simulink library "BLDC"  (R2012b)
settings: Solver=ode45  StartTime=0.0  StopTime=10.0  RelTol=1e-3
undefined symbols (not defined in the file): fcem_a, fcem_b, fcem_c
libraries: simulink x30, Tools x6
settings Model: Creator=Juliano  LastModifiedBy=h3now

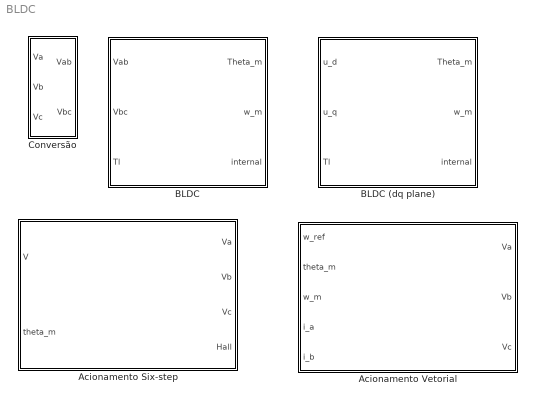
== system BLDC ==
  Acionamento Six-step : Subsystem  mask(Acionamento six-step){P=8}
      mask prompts: P "Número de pólos do motor"
      mask help:
      | Entradas
      | - V: Tensão que será aplicada nas bobinas quando forem comutadas [V]
      | - theta_m: Posição angular do rotor [rad]
      |
      | Saídas
      | - Va: Tensão que deverá ser aplicada na fase a do motor [V]
      | - Vb: Tensão que deverá ser aplicada na fase b do motor [V]
      | - Vc: Tensão que deverá ser aplicada na fase c do motor [V]
      | - Hall: Vetor 3x1 com os sinais logicos de cada sensor hall
  Acionamento Vetorial : Subsystem  mask(Acionamento Vetorial){P=8}
      mask prompts: P "Número de pólos do motor"
      mask help:
      | Entradas
      | - w_ref: Velocidade angular de referência [rpm]
      | - theta_m: Posição angular do rotor [rad]
      | - w_m: Velocidade angular do rotor [rad/s]
      | - i_a: Corrente da fase 'a' do BDLC [A]
      | - i_b: Corrente da fase 'b' do BLDC [A]
      |
      | Saídas
      | - Va: Tensão que deverá ser aplicada na fase a do motor [V]
      | - Vb: Tensão que deverá ser aplicada na fase b do motor [V]
      | - Vc: Tensão que deverá ser aplicada na fase c do motor [V]
  BLDC : Subsystem  mask(Simulador de um motor BLDC){J=1.39e-6, R=10.1/2, L=2.04/2000, P=8, Kt=15.7e-3/1.19, Ke=15.7e-3/1.19, Kd=0, F_stick=0, F_slip=0, default_fcem=on, fcem_a=fcem_a, fcem_b=fcem_b, fcem_c=fcem_c}
      mask prompts: J "Inércia do sistema motor+carga [Kg.m^2]"; R "Resistência por fase [Ohm]"; L "Indutância por fase (descontado o valor da indutância mútua, se for significativo) [Henry]"; P "Número de pólos"; Kt "Constante de torque [Nm/A]"; Ke "Constante de força eletromotriz [V.s] (numericamente igual à constante de torque se utilizar SI)"; Kd "Constante de atrito viscoso"; F_stick "Força máxima de atrito estático"; F_slip "Força de atrito dinâmico"; default_fcem "Utilizar back-emf trapezoidal?"; fcem_a "Lookup table da back-emf fase a"; fcem_b "Lookup table da back-emf fase b"; fcem_c "Lookup table da back-emf fase c"
      mask help:
      | Entradas
      | - Vab: Diferença de potencial entre a fase 'a' e a fase 'b' [V]
      | - Vbc: Diferença de potencial entre a fase 'b' e a fase 'c' [V]
      | - Tl: torque da carga [N.m]
      |
      | Saídas
      | - Theta_m: ângulo do rotor [rad]
      | - w_m: velocidade ângular do rotor [rad/s]
      | - internal: vetor de variáveis internas do simulador:
      |     - FCEM em cada fase [V] (3x1)
      |     - Corrente em cada fase [A] (3x1)
      |     - Torque produzido por cada fase [N.m] (3x1)
      |     - Torque total [N.m] (1x1)
      |     - Torque de atrito [N.m] (1x1)
      mask init:
      | % Se o usuário escolheu utilizar a back-emf padrão, inicializa as variáveis
      | % da lookuptables com valores zerados para não dar erro.
      | if default_fcem == 1
      |     fcem_a = [0,0;1,0];
      |     fcem_b = [0,0;1,0];
      |     fcem_c = [0,0;1,0];
      |     
      | % Se o usuário escolheu especificar qual será a forma da back-emf, checa se
      | % as lookup tables que ele inseriu fazem sentido.
      | else
      |     % Checa se a primeira coluna começa em 0.
      |     if fcem_a(1,1) ~= 0 ||fcem_b(1,1) ~= 0 || fcem_c(1,1) ~= 0
      |         error('A primeira coluna das lookup tables que definem o formato da back-emf devem começar em zero!');
      |     end
      |     % Checa se a primeira coluna termina em 360.
      |     if fcem_a(size(fcem_a,1),1) ~= 360 || fcem_b(size(fcem_b,1),1) ~= 360 || fcem_c(size(fcem_c,1),1) ~= 360
      |         error('A primeira coluna das lookup tables que definem o formato da back-emf deve terminar em 360!');
      |     end
      | end
      mask TypeOptions F_stick: Dinâmica mecânica /Atrito de coulomb/F_stick
      mask TypeOptions F_slip: Dinâmica mecânica /Atrito de coulomb/F_slip
      mask Callback default_fcem:
      | maskStr = get_param(gcb,'MaskValues');
      | 
      | if strcmp(maskStr{10},'on')
      |     set_param(gcb,'MaskVisibilities',{'on';'on';'on';'on';'on';'on';'on';'on';'on';'on';'off';'off';'off'});
      | else
      |     set_param(gcb,'MaskVisibilities',{'on';'on';'on';'on';'on';'on';'on';'on';'on';'on';'on';'on';'on'});
      | end
  BLDC (dq plane) : Subsystem  mask(BLDC Simulator (in dq space coordinates)){J=1.39e-6, R=10.1/2, L=2.04/2000, P=8, Kt=15.7e-3/1.19, Ke=15.7e-3/1.19, Kd=0, F_stick=0, F_slip=0, default_fcem=on, fcem_a=0, fcem_b=0, fcem_c=0}
      mask prompts: J "Inércia do sistema motor+carga [Kg.m^2]"; R "Resistência por Fase [Ohm]"; L "Indutância por fase (descontado o valor da indutância mútua, se for significativo) [Henry]"; P "Número de pólos"; Kt "Constante de torque [N.m/A]"; Ke "Constante de força eletromotriz [V.s]"; Kd "Constante de atrito viscoso"; F_stick "Torque máximo de atrito estático [N.m]"; F_slip "Torque de atrito dinâmico [N.m]"; default_fcem "Utilizar back-emf padrão?"; fcem_a "Forma da back-emf na fase a"; fcem_b "Forma da back-emf na fase b"; fcem_c "Forma da back-emf na fase c"
      mask help:
      | Entradas
      | - u_d: D component of the Vabc voltages projection in the dq plane [V]
      | - u_q: Q component of the Vabc voltages projection in the dq plane [V]
      | - Tl: Load torque [N.m]
      |
      | Saídas
      | - Theta_m: Rotor angle [rad]
      | - w_m: Rotor angular velocity [rad/s]
      | - internal: Vector of internal variables from the simulator:
      |     - Electrical torque: The electrical torque generated by the BLDC
      |     - Currents [2x1]
      |         - i_d: D component of the i_abc currents projection in the dq plane.
      |         - i_q: Q component of the i_abc currents projection in the dq plane.
      |     - Back emfs [2x1]
      |         - e_d: D component of the e_abc back-emfs projection in the dq plane.
      |         - e_q: Q component of the e_abc back_emfs projection in the dq plane.
      |     - Friction Torque: The friction torque acting in the rotor.
      mask init: same as BLDC/BLDC
      mask TypeOptions F_stick: Mechanical model/Atrito de coulomb/F_stick
      mask TypeOptions F_slip: Mechanical model/Atrito de coulomb/F_slip
      mask Callback default_fcem:
      | maskStr = get_param(gcb,'MaskValues');
      | 
      | if strcmp(maskStr{10},'on')
      |     set_param(gcb,'MaskVisibilities',{'on';'on';'on';'on';'on';'on';'on';'on';'on';'on';'off';'off';'off'});
      | else
      |     set_param(gcb,'MaskVisibilities',{'on';'on';'on';'on';'on';'on';'on';'on';'on';'on';'on';'on';'on'});
      | end
  Conversão : Subsystem

== system BLDC/Acionamento Six-step ==
  V : Inport
  theta_m : Inport  Port=2
  Anti-horário : Constant
  Data Type Conversion3 : DataTypeConversion  SaturateOnIntegerOverflow=on  RndMeth=Zero
  Decoder : Subsystem
  Gain : Gain  Gain=P/2
  Inversor : Subsystem
  Sensores Hall : Subsystem
  Va : Outport
  Vb : Outport  Port=2
  Vc : Outport  Port=3
  Hall : Outport  Port=4
  wires:
  theta_m/1 -> Gain/1
  Gain/1 -> Sensores Hall/1(teta_e)
  Decoder/1(Gates) -> Inversor/1(Gates)
  Anti-horário/1 -> Decoder/2(Sentido de rotação)
  V/1 -> Inversor/2(Vcc)
  Sensores Hall/1(Hall) -> Hall/1, Data Type Conversion3/1  "Hall"
  Data Type Conversion3/1 -> Decoder/1("Hall ")
  Inversor/1(Va) -> Va/1
  Inversor/2(Vb) -> Vb/1
  Inversor/3(Vc) -> Vc/1

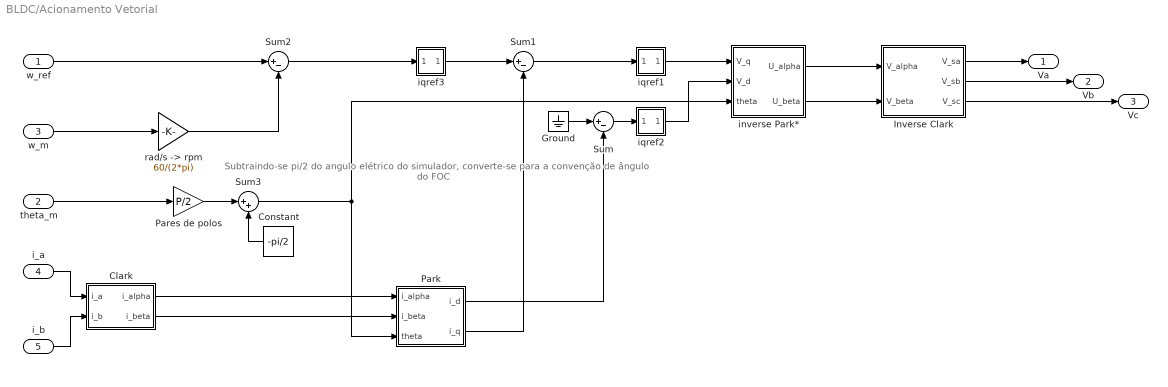
== system BLDC/Acionamento Vetorial ==
  note: Subtraindo-se pi/2 do angulo elétrico
      | do simulador, converte-se para a
      | convenção de ângulo do FOC
  w_ref : Inport
  theta_m : Inport  Port=2
  w_m : Inport  Port=3
  i_a : Inport  Port=4
  i_b : Inport  Port=5
  Clark : Subsystem
  Constant : Constant  Value=-pi/2
  Ground : Ground
  Inverse Clark : Subsystem
  Pares de polos : Gain  Gain=P/2
  Park : Subsystem
  Sum : Sum  Inputs=|+-
  Sum1 : Sum  Inputs=|+-
  Sum2 : Sum  Inputs=|+-
  Sum3 : Sum  Inputs=|++
  inverse Park* : Subsystem
  iqref1 : Subsystem  mask(PI Controller){I=0.5, P=1, sat=[-500, 500]}
      mask prompts: I "Integral"; P "Proportional:"; sat "Minimum and maximum outputs:"
      mask init:
      | min=sat(1);max=sat(2);
      mask Display: disp('PI')
  iqref2 : Subsystem  mask(PI Controller){I=5, P=10, sat=[-500, 500]}
      mask prompts: I "Integral"; P "Proportional:"; sat "Minimum and maximum outputs:"
      mask init:
      | min=sat(1);max=sat(2);
      mask Display: disp('PI')
  iqref3 : Subsystem  mask(PI Controller){I=0.1, P=0.1, sat=[-500, 500]}
      mask prompts: I "Integral"; P "Proportional:"; sat "Minimum and maximum outputs:"
      mask init:
      | min=sat(1);max=sat(2);
      mask Display: disp('PI')
  "rad/s -> rpm" : Gain  Gain=60/(2*pi)
  Va : Outport
  Vb : Outport  Port=2
  Vc : Outport  Port=3
  wires:
  theta_m/1 -> Pares de polos/1
  Pares de polos/1 -> Sum3/1
  Constant/1 -> Sum3/2
  w_ref/1 -> Sum2/1
  i_b/1 -> Clark/2(i_b)
  Sum1/1 -> iqref1/1(In_1)
  Inverse Clark/2(V_sb) -> Vb/1
  Sum2/1 -> iqref3/1(In_1)
  iqref3/1(Out_1) -> Sum1/1
  Inverse Clark/1(V_sa) -> Va/1
  Inverse Clark/3(V_sc) -> Vc/1
  i_a/1 -> Clark/1(i_a)
  iqref1/1(Out_1) -> inverse Park*/1(V_q)
  "rad/s -> rpm"/1 -> Sum2/2
  Park/2(i_q) -> Sum1/2
  Sum3/1 -> inverse Park*/3(theta), Park/3(theta)
  iqref2/1(Out_1) -> inverse Park*/2(V_d)
  w_m/1 -> "rad/s -> rpm"/1
  Ground/1 -> Sum/1
  Park/1(i_d) -> Sum/2
  Sum/1 -> iqref2/1(In_1)
  Clark/2(i_beta) -> Park/2(i_beta)
  Clark/1(i_alpha) -> Park/1(i_alpha)
  inverse Park*/1(U_alpha) -> Inverse Clark/1(V_alpha)
  inverse Park*/2(U_beta) -> Inverse Clark/2(V_beta)

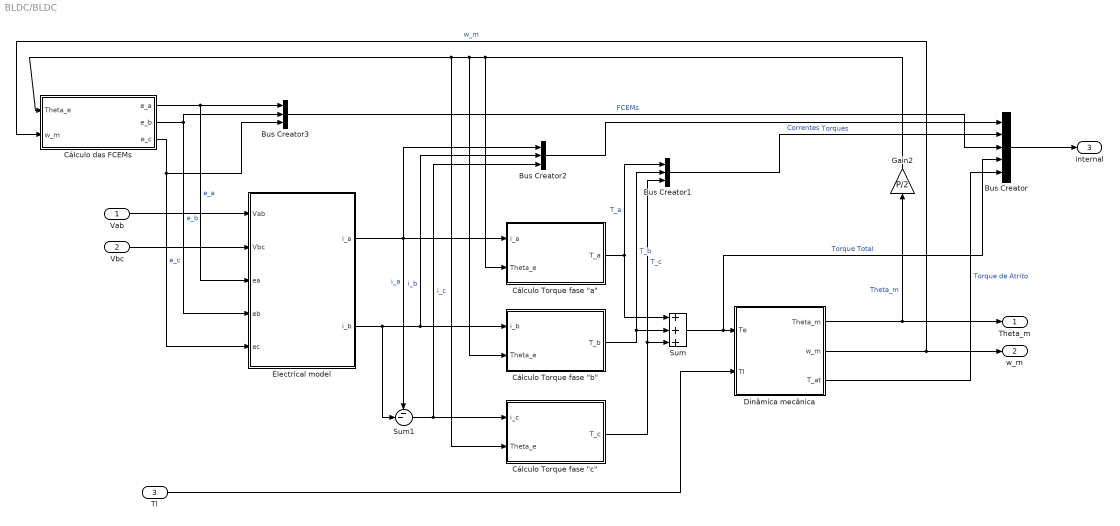
== system BLDC/BLDC ==
  Vab : Inport
  Vbc : Inport  Port=2
  Tl : Inport  Port=3
  Bus Creator : BusCreator  Inputs=5
  Bus Creator1 : BusCreator  Inputs=3
  Bus Creator2 : BusCreator  Inputs=3
  Bus Creator3 : BusCreator  Inputs=3
  "Cálculo Torque fase \"a\"" : Subsystem
  "Cálculo Torque fase \"b\"" : Subsystem
  "Cálculo Torque fase \"c\"" : Subsystem
  Cálculo das FCEMs : Subsystem
  "Dinâmica mecânica " : Subsystem
  Electrical model : Subsystem
  Gain2 : Gain  Gain=P/2
  Sum : Sum  Inputs=+++
  Sum1 : Sum  Inputs=--|
  Theta_m : Outport
  w_m : Outport  Port=2
  internal : Outport  Port=3
  wires:
  Gain2/1 -> "Cálculo Torque fase \"b\""/2(Theta_e), Cálculo das FCEMs/1(Theta_e), "Cálculo Torque fase \"c\""/2(Theta_e), "Cálculo Torque fase \"a\""/2(Theta_e)
  Tl/1 -> "Dinâmica mecânica "/2(Tl)
  "Dinâmica mecânica "/2(w_m) -> Cálculo das FCEMs/2(w_m), w_m/1  "w_m"
  "Dinâmica mecânica "/1(Theta_m) -> Gain2/1, Theta_m/1  "Theta_m"
  Sum/1 -> Bus Creator/4, "Dinâmica mecânica "/1(Te)  "Torque Total"
  "Cálculo Torque fase \"c\""/1(T_c) -> Bus Creator1/3, Sum/3  "T_c"
  "Cálculo Torque fase \"b\""/1(T_b) -> Bus Creator1/2, Sum/2  "T_b"
  "Cálculo Torque fase \"a\""/1(T_a) -> Bus Creator1/1, Sum/1  "T_a"
  Sum1/1 -> "Cálculo Torque fase \"c\""/1(i_c), Bus Creator2/3  "i_c"
  Electrical model/2(i_b) -> "Cálculo Torque fase \"b\""/1(i_b), Bus Creator2/2, Sum1/2  "i_b"
  Electrical model/1(i_a) -> "Cálculo Torque fase \"a\""/1(i_a), Bus Creator2/1, Sum1/1  "i_a"
  Vbc/1 -> Electrical model/2(Vbc)
  Cálculo das FCEMs/3(e_c) -> Electrical model/5(ec), Bus Creator3/3  "e_c"
  Cálculo das FCEMs/2(e_b) -> Electrical model/4(eb), Bus Creator3/2  "e_b"
  Cálculo das FCEMs/1(e_a) -> Electrical model/3(ea), Bus Creator3/1  "e_a"
  Bus Creator/1 -> internal/1
  Bus Creator3/1 -> Bus Creator/3  "FCEMs"
  Bus Creator2/1 -> Bus Creator/1  "Correntes"
  Bus Creator1/1 -> Bus Creator/2  "Torques"
  Vab/1 -> Electrical model/1(Vab)
  "Dinâmica mecânica "/3(T_at) -> Bus Creator/5  "Torque de Atrito"

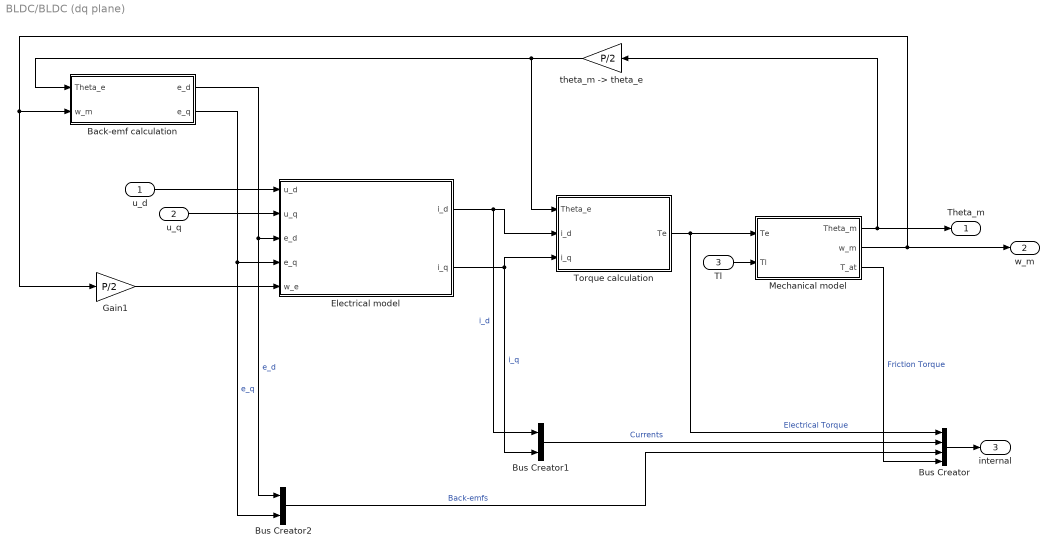
== system BLDC/BLDC (dq plane) ==
  u_d : Inport
  u_q : Inport  Port=2
  Tl : Inport  Port=3
  Back-emf calculation : Subsystem
  Bus Creator : BusCreator
  Bus Creator1 : BusCreator  Inputs=2
  Bus Creator2 : BusCreator  Inputs=2
  Electrical model : Subsystem
  Gain1 : Gain  Gain=P/2
  Mechanical model : Subsystem
  Torque calculation : Subsystem
  "theta_m -> theta_e" : Gain  Gain=P/2
  Theta_m : Outport
  w_m : Outport  Port=2
  internal : Outport  Port=3
  wires:
  Back-emf calculation/2(e_q) -> Bus Creator2/2, Electrical model/4(e_q)  "e_q"
  u_q/1 -> Electrical model/2(u_q)
  Tl/1 -> Mechanical model/2(Tl)
  Mechanical model/2(w_m) -> w_m/1, Back-emf calculation/2(w_m), Gain1/1
  Mechanical model/1(Theta_m) -> "theta_m -> theta_e"/1, Theta_m/1
  "theta_m -> theta_e"/1 -> Torque calculation/1(Theta_e), Back-emf calculation/1(Theta_e)
  Gain1/1 -> Electrical model/5(w_e)
  u_d/1 -> Electrical model/1(u_d)
  Back-emf calculation/1(e_d) -> Electrical model/3(e_d), Bus Creator2/1  "e_d"
  Electrical model/1(i_d) -> Bus Creator1/1, Torque calculation/2(i_d)  "i_d"
  Electrical model/2(i_q) -> Bus Creator1/2, Torque calculation/3(i_q)  "i_q"
  Torque calculation/1(Te) -> Bus Creator/1, Mechanical model/1(Te)  "Electrical Torque"
  Bus Creator1/1 -> Bus Creator/2  "Currents"
  Bus Creator2/1 -> Bus Creator/3  "Back-emfs"
  Bus Creator/1 -> internal/1
  Mechanical model/3(T_at) -> Bus Creator/4  "Friction Torque"

== system BLDC/Conversão ==
  Va : Inport
  Vb : Inport  Port=2
  Vc : Inport  Port=3
  Sum : Sum  Inputs=|+-
  Sum1 : Sum  Inputs=|+-
  Vab : Outport
  Vbc : Outport  Port=2
  wires:
  Va/1 -> Sum/1
  Sum/1 -> Vab/1
  Vb/1 -> Sum1/1, Sum/2
  Vc/1 -> Sum1/2
  Sum1/1 -> Vbc/1

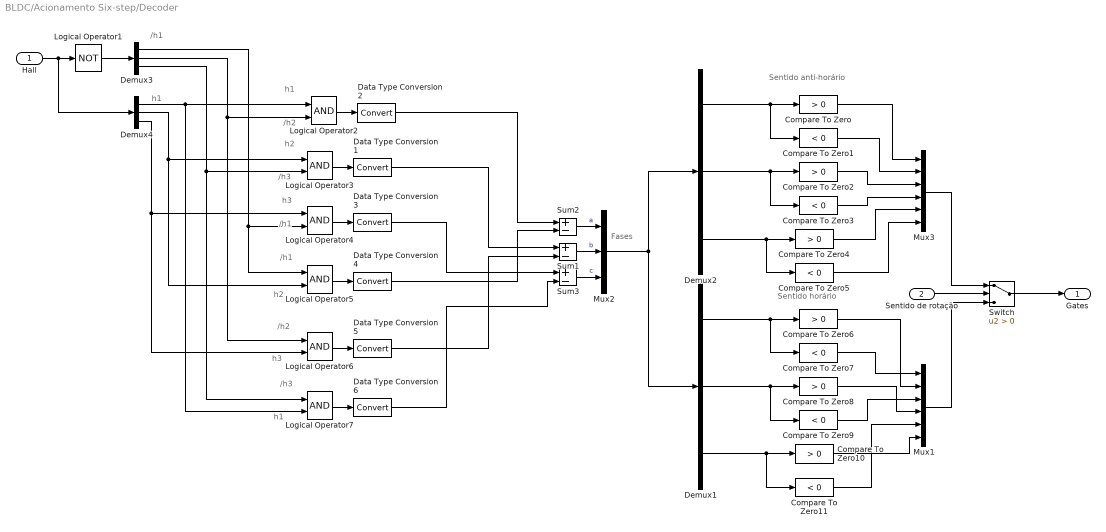
== system BLDC/Acionamento Six-step/Decoder ==
  note: Fases
  note: Sentido horário
  note: Sentido anti-horário
  note: h1
  note: /h3
  note: h3
  note: /h2
  note: h2
  note: /h1
  note: /h1
  note: h3
  note: /h3
  note: h2
  note: /h2
  note: h1
  note: h1
  note: /h1
  "Hall " : Inport
  Sentido de rotação : Inport  Port=2
  Compare To Zero{,2,4,6,8,10} (6 alike) : simulink/Logic and Bit Operations/Compare To Zero  relop=>  OutDataTypeStr=boolean  ZeroCross=off
  Compare To Zero{1,3,5,7,9,11} (6 alike) : simulink/Logic and Bit Operations/Compare To Zero  relop=<  OutDataTypeStr=boolean  ZeroCross=off
  Data Type Conversion{1..6} (6 alike) : DataTypeConversion
  Demux{1..4} (4 alike) : Demux  Outputs=3
  Logical Operator1 : Logic  Operator=NOT  AllPortsSameDT=off  OutDataTypeStr=boolean
  Logical Operator{2..7} (6 alike) : Logic  AllPortsSameDT=off  OutDataTypeStr=boolean
  Mux1 : Mux  Inputs=6
  Mux2 : Mux  Inputs=3
  Mux3 : Mux  Inputs=6
  Sum1 : Sum  Inputs=+-  OutDataTypeStr=double
  Sum2 : Sum  Inputs=+-  OutDataTypeStr=double
  Sum3 : Sum  Inputs=+-  OutDataTypeStr=double
  Switch : Switch  Criteria=u2 > Threshold
  Gates : Outport
  wires:
  Mux2/1 -> Demux1/1, Demux2/1
  Data Type Conversion6/1 -> Sum3/2
  Data Type Conversion3/1 -> Sum3/1
  Data Type Conversion5/1 -> Sum1/2
  Data Type Conversion1/1 -> Sum1/1
  Data Type Conversion4/1 -> Sum2/2
  Data Type Conversion2/1 -> Sum2/1
  Logical Operator7/1 -> Data Type Conversion6/1
  Logical Operator6/1 -> Data Type Conversion5/1
  Logical Operator5/1 -> Data Type Conversion4/1
  Logical Operator4/1 -> Data Type Conversion3/1
  Logical Operator3/1 -> Data Type Conversion1/1
  Sum3/1 -> Mux2/3  "c"
  Sum1/1 -> Mux2/2  "b"
  Sum2/1 -> Mux2/1  "a"
  Logical Operator2/1 -> Data Type Conversion2/1
  Demux3/1 -> Logical Operator5/1, Logical Operator4/2
  Demux3/2 -> Logical Operator6/1, Logical Operator2/2
  Demux3/3 -> Logical Operator7/1, Logical Operator3/2
  Demux4/1 -> Logical Operator7/2, Logical Operator2/1
  Demux4/2 -> Logical Operator5/2, Logical Operator3/1
  Demux4/3 -> Logical Operator6/2, Logical Operator4/1
  Logical Operator1/1 -> Demux3/1
  "Hall "/1 -> Demux4/1, Logical Operator1/1
  Compare To Zero10/1 -> Mux1/6
  Compare To Zero11/1 -> Mux1/5
  Compare To Zero8/1 -> Mux1/4
  Compare To Zero9/1 -> Mux1/3
  Compare To Zero6/1 -> Mux1/2
  Compare To Zero7/1 -> Mux1/1
  Switch/1 -> Gates/1
  Mux1/1 -> Switch/3
  Sentido de rotação/1 -> Switch/2
  Mux3/1 -> Switch/1
  Demux1/3 -> Compare To Zero11/1, Compare To Zero10/1
  Demux1/2 -> Compare To Zero9/1, Compare To Zero8/1
  Demux1/1 -> Compare To Zero7/1, Compare To Zero6/1
  Compare To Zero5/1 -> Mux3/6
  Compare To Zero4/1 -> Mux3/5
  Compare To Zero3/1 -> Mux3/4
  Compare To Zero2/1 -> Mux3/3
  Compare To Zero1/1 -> Mux3/2
  Compare To Zero/1 -> Mux3/1
  Demux2/3 -> Compare To Zero5/1, Compare To Zero4/1
  Demux2/2 -> Compare To Zero3/1, Compare To Zero2/1
  Demux2/1 -> Compare To Zero1/1, Compare To Zero/1

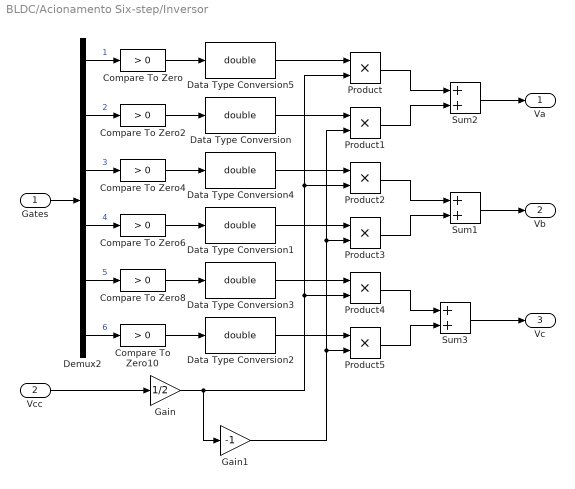
== system BLDC/Acionamento Six-step/Inversor ==
  Gates : Inport
  Vcc : Inport  Port=2
  Compare To Zero : simulink/Logic and Bit Operations/Compare To Zero  relop=>  OutDataTypeStr=uint8  ZeroCross=off
  Compare To Zero{2,6,8,10} (4 alike) : simulink/Logic and Bit Operations/Compare To Zero  relop=>  OutDataTypeStr=boolean  ZeroCross=off
  Compare To Zero4 : simulink/Logic and Bit Operations/Compare To Zero  relop=>  OutDataTypeStr=uint8  ZeroCross=off
  Data Type Conversion{,1..5} (6 alike) : DataTypeConversion  OutDataTypeStr=double
  Demux2 : Demux  Outputs=6
  Gain : Gain  Gain=1/2
  Gain1 : Gain  Gain=-1
  Product{,1..5} (6 alike) : Product  RndMeth=Zero
  Sum1 : Sum  SaturateOnIntegerOverflow=on
  Sum2 : Sum  SaturateOnIntegerOverflow=on
  Sum3 : Sum  SaturateOnIntegerOverflow=on
  Va : Outport
  Vb : Outport  Port=2
  Vc : Outport  Port=3
  wires:
  Vcc/1 -> Gain/1
  Sum1/1 -> Vb/1
  Sum3/1 -> Vc/1
  Sum2/1 -> Va/1
  Gates/1 -> Demux2/1
  Demux2/1 -> Compare To Zero/1  "1"
  Demux2/2 -> Compare To Zero2/1  "2"
  Demux2/3 -> Compare To Zero4/1  "3"
  Demux2/4 -> Compare To Zero6/1  "4"
  Demux2/5 -> Compare To Zero8/1  "5"
  Demux2/6 -> Compare To Zero10/1  "6"
  Compare To Zero/1 -> Data Type Conversion5/1
  Compare To Zero2/1 -> Data Type Conversion/1
  Compare To Zero4/1 -> Data Type Conversion4/1
  Compare To Zero6/1 -> Data Type Conversion1/1
  Compare To Zero8/1 -> Data Type Conversion3/1
  Compare To Zero10/1 -> Data Type Conversion2/1
  Product/1 -> Sum2/1
  Product1/1 -> Sum2/2
  Product2/1 -> Sum1/1
  Product3/1 -> Sum1/2
  Product4/1 -> Sum3/1
  Product5/1 -> Sum3/2
  Data Type Conversion2/1 -> Product5/1
  Data Type Conversion3/1 -> Product4/1
  Data Type Conversion1/1 -> Product3/1
  Data Type Conversion4/1 -> Product2/1
  Data Type Conversion/1 -> Product1/1
  Data Type Conversion5/1 -> Product/1
  Gain1/1 -> Product5/2, Product3/2, Product1/2
  Gain/1 -> Gain1/1, Product4/2, Product2/2, Product/2

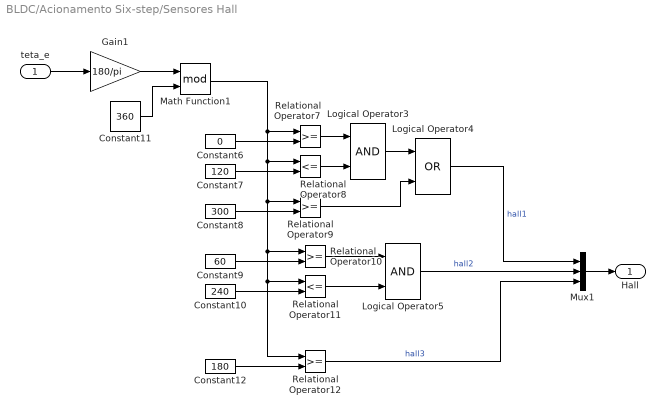
== system BLDC/Acionamento Six-step/Sensores Hall ==
  teta_e : Inport
  Constant10 : Constant  Value=240
  Constant11 : Constant  Value=360
  Constant12 : Constant  Value=180
  Constant6 : Constant  Value=0
  Constant7 : Constant  Value=120
  Constant8 : Constant  Value=300
  Constant9 : Constant  Value=60
  Gain1 : Gain  Gain=180/pi
  Logical Operator3 : Logic  AllPortsSameDT=off  OutDataTypeStr=boolean
  Logical Operator4 : Logic  Operator=OR  AllPortsSameDT=off  OutDataTypeStr=boolean
  Logical Operator5 : Logic  AllPortsSameDT=off  OutDataTypeStr=boolean
  Math Function1 : Math  Operator=mod  SaturateOnIntegerOverflow=on
  Mux1 : Mux  Inputs=3
  Relational Operator{7,9..10,12} (4 alike) : RelationalOperator  InputSameDT=on
  Relational Operator11 : RelationalOperator  Operator=<=  InputSameDT=on
  Relational Operator8 : RelationalOperator  Operator=<=  InputSameDT=on
  Hall : Outport
  wires:
  teta_e/1 -> Gain1/1
  Constant6/1 -> Relational Operator7/2
  Constant7/1 -> Relational Operator8/2
  Constant8/1 -> Relational Operator9/2
  Relational Operator9/1 -> Logical Operator4/2
  Logical Operator3/1 -> Logical Operator4/1
  Relational Operator7/1 -> Logical Operator3/1
  Relational Operator8/1 -> Logical Operator3/2
  Relational Operator10/1 -> Logical Operator5/1
  Relational Operator11/1 -> Logical Operator5/2
  Constant9/1 -> Relational Operator10/2
  Constant10/1 -> Relational Operator11/2
  Constant12/1 -> Relational Operator12/2
  Mux1/1 -> Hall/1
  Logical Operator4/1 -> Mux1/1  "hall1"
  Logical Operator5/1 -> Mux1/2  "hall2"
  Relational Operator12/1 -> Mux1/3  "hall3"
  Gain1/1 -> Math Function1/1
  Constant11/1 -> Math Function1/2
  Math Function1/1 -> Relational Operator8/1, Relational Operator9/1, Relational Operator10/1, Relational Operator11/1, Relational Operator12/1, Relational Operator7/1

== system BLDC/Acionamento Vetorial/Clark ==
  i_a : Inport
  i_b : Inport  Port=2
  Add : Sum
  Gain : Gain  Gain=2
  Gain1 : Gain  Gain=1/sqrt(3)
  i_alpha : Outport
  i_beta : Outport  Port=2
  wires:
  Gain1/1 -> i_beta/1
  Add/1 -> Gain1/1
  Gain/1 -> Add/2
  i_b/1 -> Gain/1
  i_a/1 -> Add/1, i_alpha/1

== system BLDC/Acionamento Vetorial/Inverse Clark ==
  V_alpha : Inport
  V_beta : Inport  Port=2
  Add : Sum  Inputs=-+
  Add1 : Sum  Inputs=--
  Gain : Gain  Gain=0.5
  Gain1 : Gain  Gain=sqrt(3)
  Gain2 : Gain  Gain=0.5
  V_sa : Outport
  V_sb : Outport  Port=2
  V_sc : Outport  Port=3
  wires:
  Gain1/1 -> Add1/1, Add/2
  V_beta/1 -> Gain1/1
  Gain2/1 -> V_sc/1
  Add1/1 -> Gain2/1
  Gain/1 -> V_sb/1
  Add/1 -> Gain/1
  V_alpha/1 -> V_sa/1, Add1/2, Add/1

== system BLDC/Acionamento Vetorial/Park ==
  i_alpha : Inport
  i_beta : Inport  Port=2
  theta : Inport  Port=3
  Add : Sum
  Add1 : Sum  Inputs=-+
  Product : Product  RndMeth=Zero
  Product1 : Product  RndMeth=Zero
  Trigonometric Function : Trigonometry  OutputSignalType=real
  Trigonometric Function1 : Trigonometry  Operator=cos  OutputSignalType=real
  i_d : Outport
  i_q : Outport  Port=2
  wires:
  Add1/1 -> i_q/1
  Product1/1 -> Add1/2, Add/2
  Product/1 -> Add1/1, Add/1
  i_alpha/1 -> Product1/2
  Trigonometric Function1/1 -> Product1/1
  Add/1 -> i_d/1
  Trigonometric Function/1 -> Product/2
  i_beta/1 -> Product/1
  theta/1 -> Trigonometric Function1/1, Trigonometric Function/1

== system BLDC/Acionamento Vetorial/inverse Park* ==
  note: U_alpha = V_d*cos(theta) - V_q*sin(theta)
      | U_beta = V_d*sin(theta) + V_q*cos(theta)
  V_q : Inport
  V_d : Inport  Port=2
  theta : Inport  Port=3
  Add : Sum
  Add1 : Sum  Inputs=-+
  Gain : Gain
  Gain1 : Gain
  Product{,1..3} (4 alike) : Product  RndMeth=Zero
  Trigonometric Function : Trigonometry  OutputSignalType=real
  Trigonometric Function1 : Trigonometry  Operator=cos  OutputSignalType=real
  U_alpha : Outport
  U_beta : Outport  Port=2
  wires:
  Gain1/1 -> U_alpha/1
  Add1/1 -> Gain1/1
  Gain/1 -> U_beta/1
  Add/1 -> Gain/1
  Product3/1 -> Add1/1
  Product2/1 -> Add1/2
  Product1/1 -> Add/2
  Product/1 -> Add/1
  Trigonometric Function/1 -> Product3/1, Product1/1
  V_d/1 -> Product2/2, Product1/2
  Trigonometric Function1/1 -> Product2/1, Product/2
  V_q/1 -> Product3/2, Product/1
  theta/1 -> Trigonometric Function/1, Trigonometric Function1/1

== system BLDC/Acionamento Vetorial/iqref1 ==
  In_1 : Inport
  Integral : TransferFcn  Numerator=[I]  Denominator=[1 0]
  Proportional : Gain  Gain=P  SaturateOnIntegerOverflow=on  OutDataTypeStr=Inherit: Same as input  ParamDataTypeStr=Inherit: Same as input
  Saturation : Saturate  UpperLimit=max  LowerLimit=min
  Sum : Sum  SaturateOnIntegerOverflow=on  InputSameDT=on  OutDataTypeStr=Inherit: Same as first input
  Out_1 : Outport  InitialOutput=0
  wires:
  Integral/1 -> Sum/2
  In_1/1 -> Integral/1, Proportional/1
  Proportional/1 -> Sum/1
  Sum/1 -> Saturation/1
  Saturation/1 -> Out_1/1

== system BLDC/Acionamento Vetorial/iqref2 ==
  In_1 : Inport
  Integral : TransferFcn  Numerator=[I]  Denominator=[1 0]
  Proportional : Gain  Gain=P  SaturateOnIntegerOverflow=on  OutDataTypeStr=Inherit: Same as input  ParamDataTypeStr=Inherit: Same as input
  Saturation : Saturate  UpperLimit=max  LowerLimit=min
  Sum : Sum  SaturateOnIntegerOverflow=on  InputSameDT=on  OutDataTypeStr=Inherit: Same as first input
  Out_1 : Outport  InitialOutput=0
  wires:
  Integral/1 -> Sum/2
  In_1/1 -> Integral/1, Proportional/1
  Proportional/1 -> Sum/1
  Sum/1 -> Saturation/1
  Saturation/1 -> Out_1/1

== system BLDC/Acionamento Vetorial/iqref3 ==
  In_1 : Inport
  Integral : TransferFcn  Numerator=[I]  Denominator=[1 0]
  Proportional : Gain  Gain=P  SaturateOnIntegerOverflow=on  OutDataTypeStr=Inherit: Same as input  ParamDataTypeStr=Inherit: Same as input
  Saturation : Saturate  UpperLimit=max  LowerLimit=min
  Sum : Sum  SaturateOnIntegerOverflow=on  InputSameDT=on  OutDataTypeStr=Inherit: Same as first input
  Out_1 : Outport  InitialOutput=0
  wires:
  Integral/1 -> Sum/2
  In_1/1 -> Proportional/1, Integral/1
  Proportional/1 -> Sum/1
  Sum/1 -> Saturation/1
  Saturation/1 -> Out_1/1

== system BLDC/BLDC/Cálculo Torque fase "a" ==
  i_a : Inport
  Theta_e : Inport  Port=2
  Constant1 : Constant  Value=360
  Gain : Gain  Gain=Kt/2
  Gain1 : Gain  Gain=180/pi
  Math Function1 : Math  Operator=mod  SaturateOnIntegerOverflow=on
  Product : Product  RndMeth=Zero
  forma back-emf a : Subsystem
  T_a : Outport
  wires:
  Constant1/1 -> Math Function1/2
  Gain1/1 -> Math Function1/1
  Product/1 -> T_a/1
  forma back-emf a/1(e_a) -> Product/1
  Theta_e/1 -> Gain1/1
  Math Function1/1 -> forma back-emf a/1(theta)
  Gain/1 -> Product/2
  i_a/1 -> Gain/1

== system BLDC/BLDC/Cálculo Torque fase "b" ==
  i_b : Inport
  Theta_e : Inport  Port=2
  Constant1 : Constant  Value=360
  Gain : Gain  Gain=Kt/2
  Gain1 : Gain  Gain=180/pi
  Math Function1 : Math  Operator=mod  SaturateOnIntegerOverflow=on
  Product : Product  RndMeth=Zero
  forma back-emf b : Subsystem
  T_b : Outport
  wires:
  Constant1/1 -> Math Function1/2
  Gain1/1 -> Math Function1/1
  i_b/1 -> Gain/1
  Gain/1 -> Product/2
  Math Function1/1 -> forma back-emf b/1(theta)
  Theta_e/1 -> Gain1/1
  forma back-emf b/1(e_b) -> Product/1
  Product/1 -> T_b/1

== system BLDC/BLDC/Cálculo Torque fase "c" ==
  i_c : Inport
  Theta_e : Inport  Port=2
  Constant1 : Constant  Value=360
  Gain : Gain  Gain=Kt/2
  Gain1 : Gain  Gain=180/pi
  Math Function1 : Math  Operator=mod  SaturateOnIntegerOverflow=on
  Product : Product  RndMeth=Zero
  forma back-emf c : Subsystem
  T_c : Outport
  wires:
  Constant1/1 -> Math Function1/2
  Gain1/1 -> Math Function1/1
  Product/1 -> T_c/1
  forma back-emf c/1(e_c) -> Product/1
  Theta_e/1 -> Gain1/1
  Math Function1/1 -> forma back-emf c/1(theta)
  Gain/1 -> Product/2
  i_c/1 -> Gain/1

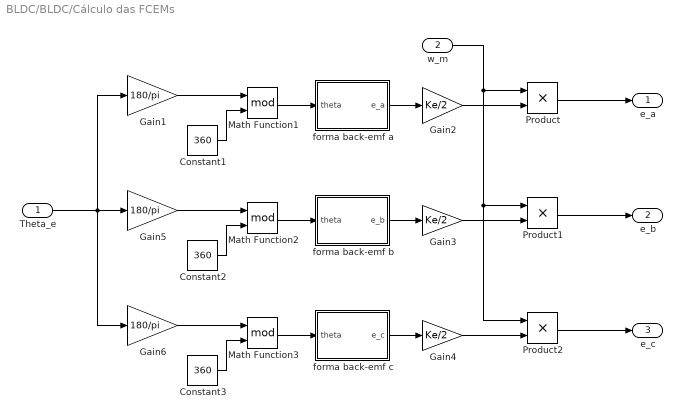
== system BLDC/BLDC/Cálculo das FCEMs ==
  Theta_e : Inport
  w_m : Inport  Port=2
  Constant1 : Constant  Value=360
  Constant2 : Constant  Value=360
  Constant3 : Constant  Value=360
  Gain1 : Gain  Gain=180/pi
  Gain2 : Gain  Gain=Ke/2
  Gain3 : Gain  Gain=Ke/2
  Gain4 : Gain  Gain=Ke/2
  Gain5 : Gain  Gain=180/pi
  Gain6 : Gain  Gain=180/pi
  Math Function1 : Math  Operator=mod  SaturateOnIntegerOverflow=on
  Math Function2 : Math  Operator=mod  SaturateOnIntegerOverflow=on
  Math Function3 : Math  Operator=mod  SaturateOnIntegerOverflow=on
  Product : Product  RndMeth=Zero
  Product1 : Product  RndMeth=Zero
  Product2 : Product  RndMeth=Zero
  forma back-emf a : Subsystem
  forma back-emf b : Subsystem
  forma back-emf c : Subsystem
  e_a : Outport
  e_b : Outport  Port=2
  e_c : Outport  Port=3
  wires:
  Constant3/1 -> Math Function3/2
  Constant2/1 -> Math Function2/2
  Constant1/1 -> Math Function1/2
  Product/1 -> e_a/1
  Product1/1 -> e_b/1
  Theta_e/1 -> Gain5/1, Gain1/1, Gain6/1
  Product2/1 -> e_c/1
  Gain2/1 -> Product/2
  w_m/1 -> Product/1, Product1/1, Product2/1
  Gain3/1 -> Product1/2
  Gain4/1 -> Product2/2
  Gain1/1 -> Math Function1/1
  Gain5/1 -> Math Function2/1
  Gain6/1 -> Math Function3/1
  Math Function1/1 -> forma back-emf a/1(theta)
  forma back-emf a/1(e_a) -> Gain2/1
  Math Function2/1 -> forma back-emf b/1(theta)
  forma back-emf b/1(e_b) -> Gain3/1
  Math Function3/1 -> forma back-emf c/1(theta)
  forma back-emf c/1(e_c) -> Gain4/1

== system BLDC/BLDC/Dinâmica mecânica  ==
  Te : Inport
  Tl : Inport  Port=2
  Atrito de coulomb : Tools/Coulomb Friction  F_stick=F_stick  F_slip=F_slip
  Gain : Gain  Gain=1/J
  Gain1 : Gain  Gain=Kd
  Integrator : Integrator  ExternalReset=rising  ShowStatePort=on
  Integrator1 : Integrator
  Sum1 : Sum  Inputs=+--
  Sum2 : Sum  Inputs=+-
  Theta_m : Outport
  w_m : Outport  Port=2
  T_at : Outport  Port=3
  wires:
  Integrator1/1 -> Theta_m/1
  Tl/1 -> Sum1/2
  Gain1/1 -> Sum1/3
  Te/1 -> Sum1/1
  Integrator/1 -> Atrito de coulomb/3, w_m/1, Integrator1/1, Gain1/1
  Gain/1 -> Integrator/1
  Sum2/1 -> Gain/1
  Sum1/1 -> Sum2/1, Atrito de coulomb/1
  Atrito de coulomb/1 -> T_at/1, Sum2/2
  Atrito de coulomb/2 -> Integrator/2
  Integrator/State -> Atrito de coulomb/2

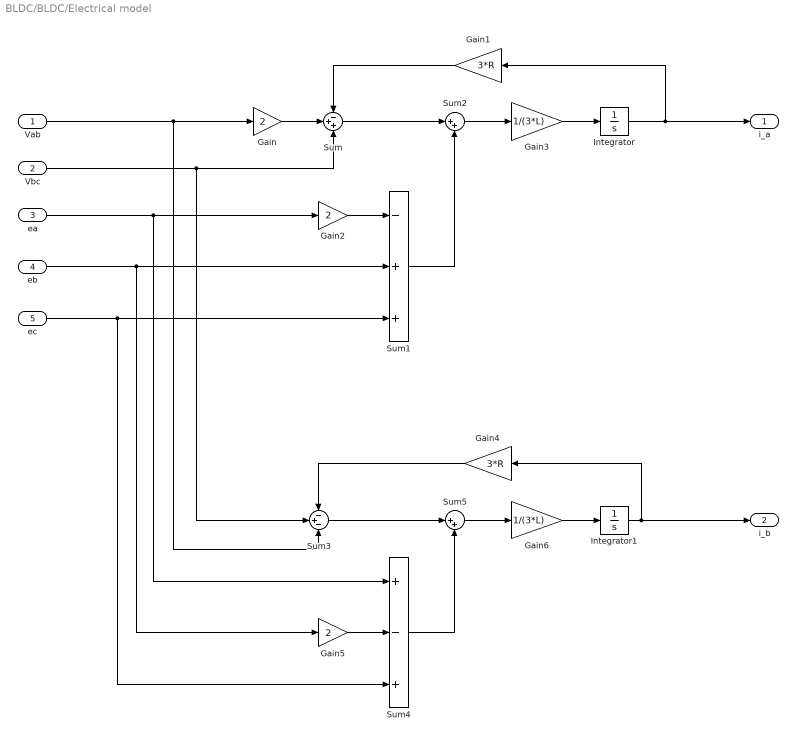
== system BLDC/BLDC/Electrical model ==
  Vab : Inport
  Vbc : Inport  Port=2
  ea : Inport  Port=3
  eb : Inport  Port=4
  ec : Inport  Port=5
  Gain : Gain  Gain=2
  Gain1 : Gain  Gain=3*R
  Gain2 : Gain  Gain=2
  Gain3 : Gain  Gain=1/(3*L)
  Gain4 : Gain  Gain=3*R
  Gain5 : Gain  Gain=2
  Gain6 : Gain  Gain=1/(3*L)
  Integrator : Integrator
  Integrator1 : Integrator
  Sum : Sum  Inputs=-++
  Sum1 : Sum  Inputs=-++
  Sum2 : Sum  Inputs=|++
  Sum3 : Sum  Inputs=-+-
  Sum4 : Sum  Inputs=+-+
  Sum5 : Sum  Inputs=|++
  i_a : Outport
  i_b : Outport  Port=2
  wires:
  Gain6/1 -> Integrator1/1
  Gain5/1 -> Sum4/2
  Sum3/1 -> Sum5/1
  Sum4/1 -> Sum5/2
  Sum5/1 -> Gain6/1
  Gain2/1 -> Sum1/1
  ea/1 -> Sum4/1, Gain2/1
  Gain1/1 -> Sum/1
  Integrator/1 -> i_a/1, Gain1/1
  Gain/1 -> Sum/2
  Vab/1 -> Sum3/3, Gain/1
  Sum2/1 -> Gain3/1
  Gain3/1 -> Integrator/1
  ec/1 -> Sum4/3, Sum1/3
  eb/1 -> Gain5/1, Sum1/2
  Sum1/1 -> Sum2/2
  Sum/1 -> Sum2/1
  Vbc/1 -> Sum3/2, Sum/3
  Gain4/1 -> Sum3/1
  Integrator1/1 -> i_b/1, Gain4/1

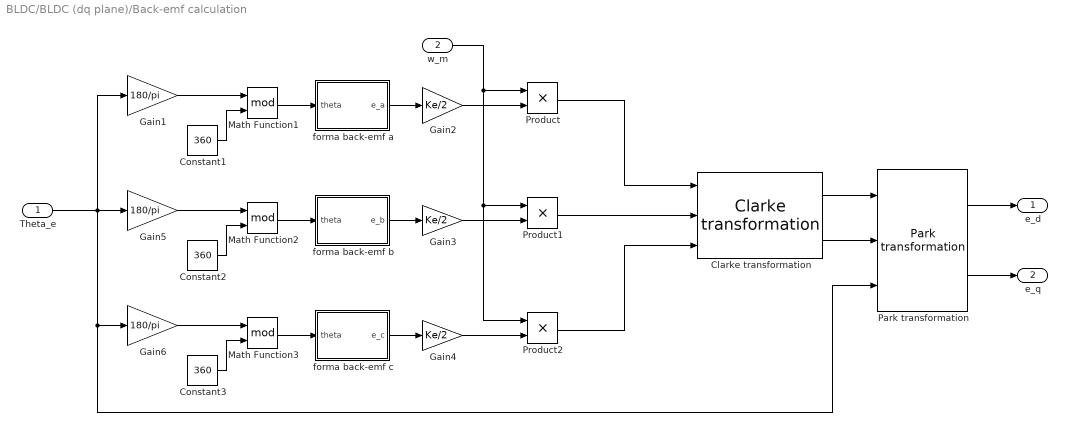
== system BLDC/BLDC (dq plane)/Back-emf calculation ==
  Theta_e : Inport
  w_m : Inport  Port=2
  Clarke transformation : Tools/Clarke transformation
  Constant1 : Constant  Value=360
  Constant2 : Constant  Value=360
  Constant3 : Constant  Value=360
  Gain1 : Gain  Gain=180/pi
  Gain2 : Gain  Gain=Ke/2
  Gain3 : Gain  Gain=Ke/2
  Gain4 : Gain  Gain=Ke/2
  Gain5 : Gain  Gain=180/pi
  Gain6 : Gain  Gain=180/pi
  Math Function1 : Math  Operator=mod  SaturateOnIntegerOverflow=on
  Math Function2 : Math  Operator=mod  SaturateOnIntegerOverflow=on
  Math Function3 : Math  Operator=mod  SaturateOnIntegerOverflow=on
  "Park transformation " : Tools/Park transformation 
  Product : Product  RndMeth=Zero
  Product1 : Product  RndMeth=Zero
  Product2 : Product  RndMeth=Zero
  forma back-emf a : Subsystem
  forma back-emf b : Subsystem
  forma back-emf c : Subsystem
  e_d : Outport
  e_q : Outport  Port=2
  wires:
  forma back-emf c/1(e_c) -> Gain4/1
  Math Function3/1 -> forma back-emf c/1(theta)
  forma back-emf b/1(e_b) -> Gain3/1
  Math Function2/1 -> forma back-emf b/1(theta)
  forma back-emf a/1(e_a) -> Gain2/1
  Math Function1/1 -> forma back-emf a/1(theta)
  Gain6/1 -> Math Function3/1
  Gain5/1 -> Math Function2/1
  Gain1/1 -> Math Function1/1
  Gain4/1 -> Product2/2
  Gain3/1 -> Product1/2
  w_m/1 -> Product2/1, Product1/1, Product/1
  Gain2/1 -> Product/2
  Product2/1 -> Clarke transformation/3
  Product1/1 -> Clarke transformation/2
  Product/1 -> Clarke transformation/1
  Constant1/1 -> Math Function1/2
  Constant2/1 -> Math Function2/2
  Constant3/1 -> Math Function3/2
  Clarke transformation/1 -> "Park transformation "/1
  Theta_e/1 -> "Park transformation "/3, Gain6/1, Gain1/1, Gain5/1
  Clarke transformation/2 -> "Park transformation "/2
  "Park transformation "/1 -> e_d/1
  "Park transformation "/2 -> e_q/1

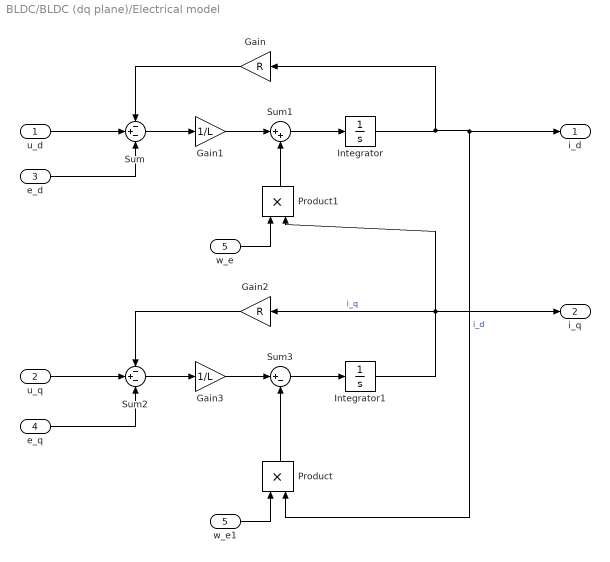
== system BLDC/BLDC (dq plane)/Electrical model ==
  u_d : Inport
  u_q : Inport  Port=2
  e_d : Inport  Port=3
  e_q : Inport  Port=4
  w_e : Inport  Port=5
  Gain : Gain  Gain=R
  Gain1 : Gain  Gain=1/L
  Gain2 : Gain  Gain=R
  Gain3 : Gain  Gain=1/L
  Integrator : Integrator
  Integrator1 : Integrator
  Product : Product  RndMeth=Zero
  Product1 : Product  RndMeth=Zero
  Sum : Sum  Inputs=-+-
  Sum1 : Sum  Inputs=|++
  Sum2 : Sum  Inputs=-+-
  Sum3 : Sum  Inputs=|+-
  w_e1 : InportShadow  Port=5
  i_d : Outport
  i_q : Outport  Port=2
  wires:
  Product/1 -> Sum3/2
  Sum3/1 -> Integrator1/1
  Gain3/1 -> Sum3/1
  Integrator1/1 -> i_q/1, Gain2/1, Product1/2  "i_q"
  Gain2/1 -> Sum2/1
  u_q/1 -> Sum2/2
  e_q/1 -> Sum2/3
  Sum2/1 -> Gain3/1
  Product1/1 -> Sum1/2
  Sum1/1 -> Integrator/1
  Integrator/1 -> i_d/1, Product/2, Gain/1  "i_d"
  e_d/1 -> Sum/3
  Gain/1 -> Sum/1
  Sum/1 -> Gain1/1
  Gain1/1 -> Sum1/1
  u_d/1 -> Sum/2
  w_e/1 -> Product1/1
  w_e1/1 -> Product/1

== system BLDC/BLDC (dq plane)/Mechanical model ==
  Te : Inport
  Tl : Inport  Port=2
  Atrito de coulomb : Tools/Coulomb Friction  F_stick=F_stick  F_slip=F_slip
  Gain : Gain  Gain=1/J
  Gain1 : Gain  Gain=Kd
  Integrator : Integrator  ExternalReset=rising  ShowStatePort=on
  Integrator1 : Integrator
  Sum1 : Sum  Inputs=+--
  Sum2 : Sum  Inputs=+-
  Theta_m : Outport
  w_m : Outport  Port=2
  T_at : Outport  Port=3
  wires:
  Integrator1/1 -> Theta_m/1
  Tl/1 -> Sum1/2
  Gain1/1 -> Sum1/3
  Te/1 -> Sum1/1
  Integrator/1 -> Atrito de coulomb/3, w_m/1, Integrator1/1, Gain1/1
  Gain/1 -> Integrator/1
  Sum2/1 -> Gain/1
  Sum1/1 -> Sum2/1, Atrito de coulomb/1
  Atrito de coulomb/1 -> T_at/1, Sum2/2
  Atrito de coulomb/2 -> Integrator/2
  Integrator/State -> Atrito de coulomb/2

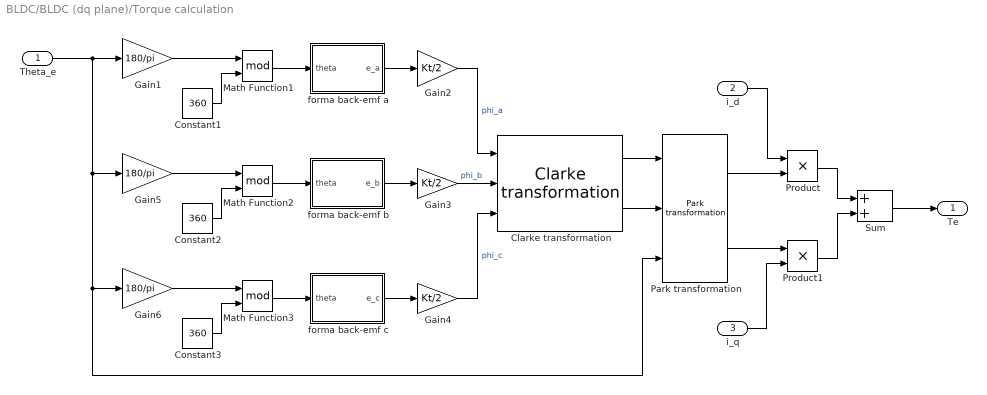
== system BLDC/BLDC (dq plane)/Torque calculation ==
  Theta_e : Inport
  i_d : Inport  Port=2
  i_q : Inport  Port=3
  Clarke transformation : Tools/Clarke transformation
  Constant1 : Constant  Value=360
  Constant2 : Constant  Value=360
  Constant3 : Constant  Value=360
  Gain1 : Gain  Gain=180/pi
  Gain2 : Gain  Gain=Kt/2
  Gain3 : Gain  Gain=Kt/2
  Gain4 : Gain  Gain=Kt/2
  Gain5 : Gain  Gain=180/pi
  Gain6 : Gain  Gain=180/pi
  Math Function1 : Math  Operator=mod  SaturateOnIntegerOverflow=on
  Math Function2 : Math  Operator=mod  SaturateOnIntegerOverflow=on
  Math Function3 : Math  Operator=mod  SaturateOnIntegerOverflow=on
  "Park transformation " : Tools/Park transformation 
  Product : Product  RndMeth=Zero
  Product1 : Product  RndMeth=Zero
  Sum : Sum
  forma back-emf a : Subsystem
  forma back-emf b : Subsystem
  forma back-emf c : Subsystem
  Te : Outport
  wires:
  forma back-emf c/1(e_c) -> Gain4/1
  Math Function3/1 -> forma back-emf c/1(theta)
  forma back-emf b/1(e_b) -> Gain3/1
  Math Function2/1 -> forma back-emf b/1(theta)
  forma back-emf a/1(e_a) -> Gain2/1
  Math Function1/1 -> forma back-emf a/1(theta)
  Gain6/1 -> Math Function3/1
  Gain5/1 -> Math Function2/1
  Gain1/1 -> Math Function1/1
  Gain4/1 -> Clarke transformation/3  "phi_c"
  Gain3/1 -> Clarke transformation/2  "phi_b"
  Gain2/1 -> Clarke transformation/1  "phi_a"
  Constant1/1 -> Math Function1/2
  Constant2/1 -> Math Function2/2
  Constant3/1 -> Math Function3/2
  Theta_e/1 -> Gain6/1, "Park transformation "/3, Gain5/1, Gain1/1
  "Park transformation "/1 -> Product/2
  i_d/1 -> Product/1
  i_q/1 -> Product1/2
  "Park transformation "/2 -> Product1/1
  Product/1 -> Sum/1
  Product1/1 -> Sum/2
  Sum/1 -> Te/1
  Clarke transformation/1 -> "Park transformation "/1
  Clarke transformation/2 -> "Park transformation "/2

== system BLDC/BLDC/Cálculo Torque fase "a"/forma back-emf a ==
  theta : Inport
  1-D Lookup Table : Lookup_n-D  NumberOfTableDimensions=1  BreakpointsForDimension1=fcem_a(:,1)  Table=fcem_a(:,2)  RndMeth=Simplest  InputSameDT=on
  Compare To Zero : simulink/Logic and Bit Operations/Compare To Zero  relop=>  OutDataTypeStr=boolean
  Constant : Constant  Value=default_fcem
  Switch : Switch
  fa1 : Lookup  InputValues=[0 30 60 90 120 150 180 210 240 270 300 330 360]  Table=[ 1 1 1 0 -1 -1 -1 -1 -1 0 1 1 1]
  e_a : Outport
  wires:
  theta/1 -> 1-D Lookup Table/1, fa1/1
  Switch/1 -> e_a/1
  fa1/1 -> Switch/1
  1-D Lookup Table/1 -> Switch/3
  Compare To Zero/1 -> Switch/2
  Constant/1 -> Compare To Zero/1

== system BLDC/BLDC/Cálculo Torque fase "b"/forma back-emf b ==
  theta : Inport
  1-D Lookup Table1 : Lookup_n-D  NumberOfTableDimensions=1  BreakpointsForDimension1=fcem_b(:,1)  Table=fcem_b(:,2)  RndMeth=Simplest  InputSameDT=on
  Compare To Zero1 : simulink/Logic and Bit Operations/Compare To Zero  relop=>  OutDataTypeStr=boolean
  Constant1 : Constant  Value=default_fcem
  Switch : Switch
  fb2 : Lookup  InputValues=[0 30 60 90 120 150 180 210 240 270 300 330 360]  Table=[-1 0 1 1 1 1 1 0 -1 -1 -1 -1 -1]
  e_b : Outport
  wires:
  1-D Lookup Table1/1 -> Switch/3
  theta/1 -> 1-D Lookup Table1/1, fb2/1
  Compare To Zero1/1 -> Switch/2
  Constant1/1 -> Compare To Zero1/1
  Switch/1 -> e_b/1
  fb2/1 -> Switch/1

== system BLDC/BLDC/Cálculo Torque fase "c"/forma back-emf c ==
  theta : Inport
  1-D Lookup Table : Lookup_n-D  NumberOfTableDimensions=1  BreakpointsForDimension1=fcem_c(:,1)  Table=fcem_c(:,2)  RndMeth=Simplest  InputSameDT=on
  Compare To Zero : simulink/Logic and Bit Operations/Compare To Zero  relop=>  OutDataTypeStr=boolean
  Constant : Constant  Value=default_fcem
  Switch : Switch
  fc1 : Lookup  InputValues=[0 30 60 90 120 150 180 210 240 270 300 330 360]  Table=[-1 -1 -1 -1 -1 0 1 1 1 1 1 0 -1]
  e_c : Outport
  wires:
  1-D Lookup Table/1 -> Switch/3
  theta/1 -> 1-D Lookup Table/1, fc1/1
  Compare To Zero/1 -> Switch/2
  Constant/1 -> Compare To Zero/1
  Switch/1 -> e_c/1
  fc1/1 -> Switch/1

== system BLDC/BLDC/Cálculo das FCEMs/forma back-emf a ==
  theta : Inport
  1-D Lookup Table : Lookup_n-D  NumberOfTableDimensions=1  BreakpointsForDimension1=fcem_a(:,1)  Table=fcem_a(:,2)  RndMeth=Simplest  InputSameDT=on
  Compare To Zero : simulink/Logic and Bit Operations/Compare To Zero  relop=>  OutDataTypeStr=boolean
  Constant : Constant  Value=default_fcem
  Switch : Switch
  fa1 : Lookup  InputValues=[0 30 60 90 120 150 180 210 240 270 300 330 360]  Table=[ 1 1 1 0 -1 -1 -1 -1 -1 0 1 1 1]
  e_a : Outport
  wires:
  theta/1 -> 1-D Lookup Table/1, fa1/1
  Switch/1 -> e_a/1
  fa1/1 -> Switch/1
  1-D Lookup Table/1 -> Switch/3
  Compare To Zero/1 -> Switch/2
  Constant/1 -> Compare To Zero/1

== system BLDC/BLDC/Cálculo das FCEMs/forma back-emf b ==
  theta : Inport
  1-D Lookup Table1 : Lookup_n-D  NumberOfTableDimensions=1  BreakpointsForDimension1=fcem_b(:,1)  Table=fcem_b(:,2)  RndMeth=Simplest  InputSameDT=on
  Compare To Zero1 : simulink/Logic and Bit Operations/Compare To Zero  relop=>  OutDataTypeStr=boolean
  Constant1 : Constant  Value=default_fcem
  Switch : Switch
  fb2 : Lookup  InputValues=[0 30 60 90 120 150 180 210 240 270 300 330 360]  Table=[-1 0 1 1 1 1 1 0 -1 -1 -1 -1 -1]
  e_b : Outport
  wires:
  1-D Lookup Table1/1 -> Switch/3
  theta/1 -> 1-D Lookup Table1/1, fb2/1
  Compare To Zero1/1 -> Switch/2
  Constant1/1 -> Compare To Zero1/1
  Switch/1 -> e_b/1
  fb2/1 -> Switch/1

== system BLDC/BLDC/Cálculo das FCEMs/forma back-emf c ==
  theta : Inport
  1-D Lookup Table : Lookup_n-D  NumberOfTableDimensions=1  BreakpointsForDimension1=fcem_c(:,1)  Table=fcem_c(:,2)  RndMeth=Simplest  InputSameDT=on
  Compare To Zero : simulink/Logic and Bit Operations/Compare To Zero  relop=>  OutDataTypeStr=boolean
  Constant : Constant  Value=default_fcem
  Switch : Switch
  fc1 : Lookup  InputValues=[0 30 60 90 120 150 180 210 240 270 300 330 360]  Table=[-1 -1 -1 -1 -1 0 1 1 1 1 1 0 -1]
  e_c : Outport
  wires:
  1-D Lookup Table/1 -> Switch/3
  theta/1 -> 1-D Lookup Table/1, fc1/1
  Compare To Zero/1 -> Switch/2
  Constant/1 -> Compare To Zero/1
  Switch/1 -> e_c/1
  fc1/1 -> Switch/1

== system BLDC/BLDC (dq plane)/Back-emf calculation/forma back-emf a ==
  theta : Inport
  1-D Lookup Table : Lookup_n-D  NumberOfTableDimensions=1  BreakpointsForDimension1=fcem_a(:,1)  Table=fcem_a(:,2)  RndMeth=Simplest  InputSameDT=on
  Compare To Zero : simulink/Logic and Bit Operations/Compare To Zero  relop=>  OutDataTypeStr=boolean
  Constant : Constant  Value=default_fcem
  Switch : Switch
  fa1 : Lookup  InputValues=[0 30 60 90 120 150 180 210 240 270 300 330 360]  Table=[ 1 1 1 0 -1 -1 -1 -1 -1 0 1 1 1]
  e_a : Outport
  wires:
  Constant/1 -> Compare To Zero/1
  Compare To Zero/1 -> Switch/2
  1-D Lookup Table/1 -> Switch/3
  fa1/1 -> Switch/1
  Switch/1 -> e_a/1
  theta/1 -> fa1/1, 1-D Lookup Table/1

== system BLDC/BLDC (dq plane)/Back-emf calculation/forma back-emf b ==
  theta : Inport
  1-D Lookup Table1 : Lookup_n-D  NumberOfTableDimensions=1  BreakpointsForDimension1=fcem_b(:,1)  Table=fcem_b(:,2)  RndMeth=Simplest  InputSameDT=on
  Compare To Zero1 : simulink/Logic and Bit Operations/Compare To Zero  relop=>  OutDataTypeStr=boolean
  Constant1 : Constant  Value=default_fcem
  Switch : Switch
  fb2 : Lookup  InputValues=[0 30 60 90 120 150 180 210 240 270 300 330 360]  Table=[-1 0 1 1 1 1 1 0 -1 -1 -1 -1 -1]
  e_b : Outport
  wires:
  fb2/1 -> Switch/1
  Switch/1 -> e_b/1
  Constant1/1 -> Compare To Zero1/1
  Compare To Zero1/1 -> Switch/2
  theta/1 -> fb2/1, 1-D Lookup Table1/1
  1-D Lookup Table1/1 -> Switch/3

== system BLDC/BLDC (dq plane)/Back-emf calculation/forma back-emf c ==
  theta : Inport
  1-D Lookup Table : Lookup_n-D  NumberOfTableDimensions=1  BreakpointsForDimension1=fcem_c(:,1)  Table=fcem_c(:,2)  RndMeth=Simplest  InputSameDT=on
  Compare To Zero : simulink/Logic and Bit Operations/Compare To Zero  relop=>  OutDataTypeStr=boolean
  Constant : Constant  Value=default_fcem
  Switch : Switch
  fc1 : Lookup  InputValues=[0 30 60 90 120 150 180 210 240 270 300 330 360]  Table=[-1 -1 -1 -1 -1 0 1 1 1 1 1 0 -1]
  e_c : Outport
  wires:
  fc1/1 -> Switch/1
  Switch/1 -> e_c/1
  Constant/1 -> Compare To Zero/1
  Compare To Zero/1 -> Switch/2
  theta/1 -> fc1/1, 1-D Lookup Table/1
  1-D Lookup Table/1 -> Switch/3

== system BLDC/BLDC (dq plane)/Torque calculation/forma back-emf a ==
  theta : Inport
  1-D Lookup Table : Lookup_n-D  NumberOfTableDimensions=1  BreakpointsForDimension1=fcem_a(:,1)  Table=fcem_a(:,2)  RndMeth=Simplest  InputSameDT=on
  Compare To Zero : simulink/Logic and Bit Operations/Compare To Zero  relop=>  OutDataTypeStr=boolean
  Constant : Constant  Value=default_fcem
  Switch : Switch
  fa1 : Lookup  InputValues=[0 30 60 90 120 150 180 210 240 270 300 330 360]  Table=[ 1 1 1 0 -1 -1 -1 -1 -1 0 1 1 1]
  e_a : Outport
  wires:
  Constant/1 -> Compare To Zero/1
  Compare To Zero/1 -> Switch/2
  1-D Lookup Table/1 -> Switch/3
  fa1/1 -> Switch/1
  Switch/1 -> e_a/1
  theta/1 -> fa1/1, 1-D Lookup Table/1

== system BLDC/BLDC (dq plane)/Torque calculation/forma back-emf b ==
  theta : Inport
  1-D Lookup Table1 : Lookup_n-D  NumberOfTableDimensions=1  BreakpointsForDimension1=fcem_b(:,1)  Table=fcem_b(:,2)  RndMeth=Simplest  InputSameDT=on
  Compare To Zero1 : simulink/Logic and Bit Operations/Compare To Zero  relop=>  OutDataTypeStr=boolean
  Constant1 : Constant  Value=default_fcem
  Switch : Switch
  fb2 : Lookup  InputValues=[0 30 60 90 120 150 180 210 240 270 300 330 360]  Table=[-1 0 1 1 1 1 1 0 -1 -1 -1 -1 -1]
  e_b : Outport
  wires:
  fb2/1 -> Switch/1
  Switch/1 -> e_b/1
  Constant1/1 -> Compare To Zero1/1
  Compare To Zero1/1 -> Switch/2
  theta/1 -> fb2/1, 1-D Lookup Table1/1
  1-D Lookup Table1/1 -> Switch/3

== system BLDC/BLDC (dq plane)/Torque calculation/forma back-emf c ==
  theta : Inport
  1-D Lookup Table : Lookup_n-D  NumberOfTableDimensions=1  BreakpointsForDimension1=fcem_c(:,1)  Table=fcem_c(:,2)  RndMeth=Simplest  InputSameDT=on
  Compare To Zero : simulink/Logic and Bit Operations/Compare To Zero  relop=>  OutDataTypeStr=boolean
  Constant : Constant  Value=default_fcem
  Switch : Switch
  fc1 : Lookup  InputValues=[0 30 60 90 120 150 180 210 240 270 300 330 360]  Table=[-1 -1 -1 -1 -1 0 1 1 1 1 1 0 -1]
  e_c : Outport
  wires:
  fc1/1 -> Switch/1
  Switch/1 -> e_c/1
  Constant/1 -> Compare To Zero/1
  Compare To Zero/1 -> Switch/2
  theta/1 -> fc1/1, 1-D Lookup Table/1
  1-D Lookup Table/1 -> Switch/3
